simulink model "Rad_model"  (R2020a)
settings: Solver=VariableStepAuto  StartTime=0.0  StopTime=10.0  RelTol=1e-3
undefined symbols (not defined in the file or in its folder): paramRadarMT, phased, physconst
libraries: phaseddetectlib x5, phasedenvlib x4, phasedtxrxlib x4, simulink x1, phasedbflib x1, phasedwavlib x1, phaseddoalib x1
settings Model: Creator=saini  LastModifiedBy=saini

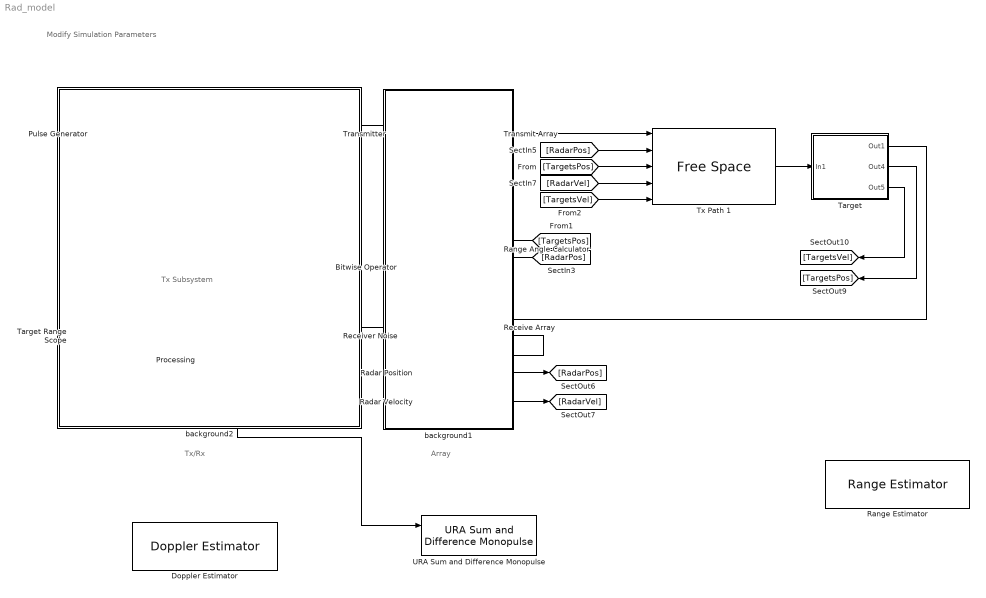
== system Rad_model ==
  note: Modify Simulation Parameters
  note: Tx/Rx
  note: Tx Subsystem
  note: Array
  Bitwise Operator : simulink/Logic and Bit Operations/Bitwise Operator  logicop=NOT  UseBitMask=off  BitMask=bin2dec('11011001')  BitMaskRealWorld=Stored Integer
  Doppler Estimator : phaseddetectlib/Doppler Estimator  NumEstimatesSource=Property  NumEstimates=1  VarianceOutputPort=off  NumPulses=2  NoisePowerSource=Property  NoisePower=1  ClusterInputPort=off  SimulateUsing=Interpreted execution
      settings: SourceProductBaseCode=AR
  Processing : Subsystem
      mask Display: disp('Signal Processing')
  Pulse Generator : phasedwavlib/Rectangular Waveform  SampleRate=paramRadarMT.fs  DurationSpecification=Pulse width  PulseWidth=1/paramRadarMT.pulseBw  DutyCycle=0.5  PRF=paramRadarMT.prf  PRFSelectionInputPort=off  SimulationTimeSource=Derive from waveform parameters  OutputFormat=Pulses  NumSamples=100  NumPulses=1  PRFOutputPort=off  SimulateUsing=Interpreted execution
      settings: SourceProductBaseCode=AR
  Radar Position : Constant  Value=[ 0; 0; 0 ]  SampleTime=1/paramRadarMT.prf
  Radar Velocity : Constant  Value=[ 0; 0; 0 ]  SampleTime=1/paramRadarMT.prf
  Range Angle Calculator : phasedenvlib/Range Angle Calculator  Model=Free space  ReferencePositionSource=Input port  ReferencePosition=[ 0; 0; 0 ]  ReferenceAxesSource=Property  ReferenceAxes=eye( 3 )  Output=Angle  SimulateUsing=Interpreted execution
      settings: SourceProductBaseCode=AR
  Range Estimator : phaseddetectlib/Range Estimator  NumEstimatesSource=Property  NumEstimates=1  VarianceOutputPort=off  RMSResolution=1  NoisePowerSource=Property  NoisePower=1  ClusterInputPort=off  SimulateUsing=Interpreted execution
      settings: SourceProductBaseCode=AR
  Receive Array : phasedtxrxlib/Narrowband Receive Array  PropagationSpeed=paramRadarMT.propSpeed  OperatingFrequency=paramRadarMT.fc  Wavefront=Plane  SensorGainMeasure=dB  Polarization=None  WeightsInputPort=off  SimulateUsing=Interpreted execution  Sensor=phased.URA('ElementSpacing',0.0150,'Size',[ 5, 5 ],'Element',phased.IsotropicAntennaElement('FrequencyRange',[ 5e9, 15e9 ]))
      settings: SourceProductBaseCode=AR
  Receiver Noise : phasedtxrxlib/Receiver Preamp  Gain=20  LossFactor=0  NoiseMethod=Noise temperature  NoiseFigure=0  ReferenceTemperature=290  SampleRateFromInputCheckbox=on  SampleRate=1e6  NoisePower=0  EnableInputPort=on  PhaseNoiseInputPort=off  SeedSource=Auto  Seed=0  SimulateUsing=Interpreted execution
      settings: SourceProductBaseCode=AR
  Target : Subsystem
      mask Display:
      | disp('Targets')
      | port_label('input',1,'X');
      | port_label('output',1,'Y');
      | port_label('output',2,'Pos');
      | port_label('output',3,'Vel');
  Target Range Scope : ArrayPlot
  Transmit Array : phasedtxrxlib/Narrowband Transmit Array  PropagationSpeed=paramRadarMT.propSpeed  OperatingFrequency=paramRadarMT.fc  CombineRadiatedSignals=on  SensorGainMeasure=dB  Polarization=None  WeightsInputPort=off  SimulateUsing=Interpreted execution  Sensor=phased.URA('Size',[ 5, 5 ],'ElementSpacing',0.0150,'Element',phased.IsotropicAntennaElement('FrequencyRange',[ 5e9, 15e9 ]))
      settings: SourceProductBaseCode=AR
  Transmitter : phasedtxrxlib/Transmitter  PeakPower=paramRadarMT.peakPower/16  Gain=paramRadarMT.txGain  LossFactor=0  InUseOutputPort=on  CoherentOnTransmit=on  PhaseNoiseOutputPort=off  SeedSource=Auto  Seed=0  SimulateUsing=Interpreted execution
      settings: SourceProductBaseCode=AR
  Tx Path 1 : phasedenvlib/Free Space  PropagationSpeed=paramRadarMT.propSpeed  OperatingFrequency=paramRadarMT.fc  TwoWayPropagation=on  SampleRateFromInputCheckbox=on  SampleRate=1e6  MaximumDistanceSource=Property  MaximumDistance=10e3  MaximumNumInputSamplesSource=Auto  MaximumNumInputSamples=1000  SimulateUsing=Interpreted execution
      settings: SourceProductBaseCode=AR
  URA Sum and Difference Monopulse : phaseddoalib/URA Sum and Difference Monopulse  PropagationSpeed=physconst( 'LightSpeed' )  OperatingFrequency=10e8  NumPhaseShifterBits=0  SimulateUsing=Interpreted execution  SensorArray=phased.URA('Element',phased.IsotropicAntennaElement('FrequencyRange',[ 5e9, 15e9 ]),'Size',[ 5, 5 ],'ElementSpacing',0.0150)
      settings: SourceProductBaseCode=AR
  background1 : Subsystem  Description=Jammer
      mask Display: disp('')
  background2 : Subsystem  Description=Jammer
      mask Display: disp('')
  wires:
  Target/1(Out1) -> Receive Array/1
  Target/3(Out5) -> [TargetsVel]
  [TargetsPos] -> Range Angle Calculator/1
  Tx Path 1/1 -> Target/1(In1)
  Target/2(Out4) -> [TargetsPos]
  [TargetsPos] -> Tx Path 1/3
  [TargetsVel] -> Tx Path 1/5
  [RadarVel] -> Tx Path 1/4
  Radar Velocity/1 -> [RadarVel]
  Transmitter/2 -> Bitwise Operator/1
  Processing/1(Out1) -> Target Range Scope/1
  Receiver Noise/1 -> URA Sum and Difference Monopulse/1, Processing/1(In1)
  Range Angle Calculator/1 -> Receive Array/2, Transmit Array/2
  Transmit Array/1 -> Tx Path 1/1
  [RadarPos] -> Range Angle Calculator/2
  [RadarPos] -> Tx Path 1/2
  Receive Array/1 -> Receiver Noise/1
  Radar Position/1 -> [RadarPos]
  Bitwise Operator/1 -> Receiver Noise/2
  Transmitter/1 -> Transmit Array/1
  Pulse Generator/1 -> Transmitter/1

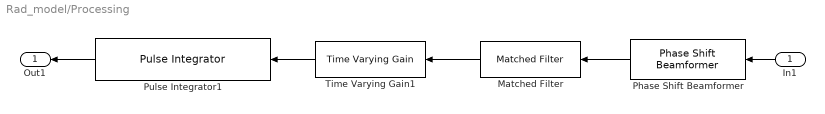
== system Rad_model/Processing ==
  In1 : Inport
  Matched Filter : phaseddetectlib/Matched Filter  CoefficientsSource=Property  Coefficients=paramRadarMT.matchingCoeff  SpectrumWindow=None  CustomSpectrumWindow=@hamming  SpectrumRange=[ 0, 1e5 ]  SampleRateFromInputCheckbox=on  SampleRate=1e6  SidelobeAttenuation=30  Beta=0.5  Nbar=4  GainOutputPort=off  MaximumNumInputSamplesSource=Auto  MaximumNumInputSamples=100  SimulateUsing=Interpreted execution
      settings: SourceProductBaseCode=AR
  Phase Shift Beamformer : phasedbflib/Phase Shift Beamformer  PropagationSpeed=paramRadarMT.propSpeed  OperatingFrequency=paramRadarMT.fc  DirectionSource=Property  Direction=[ 0; 0 ]  NumPhaseShifterBits=0  WeightsNormalization=Distortionless  WeightsOutputPort=off  SimulateUsing=Interpreted execution  SensorArray=phased.URA('ElementSpacing',0.0150,'Size',[ 5, 5 ],'Element',phased.IsotropicAntennaElement('FrequencyRange',[ 5e9, 15e9 ]))
      settings: SourceProductBaseCode=AR
  Pulse Integrator1 : phaseddetectlib/Pulse Integrator  CoherentFlag=Noncoherent  N=10  V=0
      settings: SourceProductBaseCode=AR
  Time Varying Gain1 : phaseddetectlib/Time Varying Gain  RangeLossSource=Property  RangeLoss=paramRadarMT.rangeLoss  ReferenceLoss=paramRadarMT.referenceLoss  SimulateUsing=Interpreted execution
      settings: SourceProductBaseCode=AR
  Out1 : Outport  VectorParamsAs1DForOutWhenUnconnected=off
  wires:
  Time Varying Gain1/1 -> Pulse Integrator1/1
  Matched Filter/1 -> Time Varying Gain1/1
  Pulse Integrator1/1 -> Out1/1
  In1/1 -> Phase Shift Beamformer/1
  Phase Shift Beamformer/1 -> Matched Filter/1

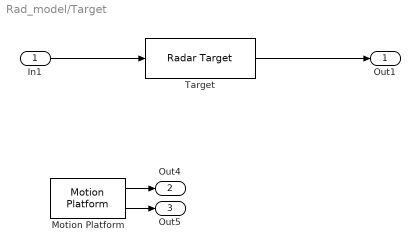
== system Rad_model/Target ==
  In1 : Inport
  Motion Platform : phasedenvlib/Motion Platform  MotionModel=Velocity  InitialPosition=paramRadarMT.targetPos  InitialVelocity=[ 0; 0; 0 ]  VelocitySource=Property  Velocity=paramRadarMT.targetVel  AccelerationSource=Property  Acceleration=[0;0;0]  CustomTrajectory=[ 0, 0, 0, 0, 0, 0, 0; 1, 0, 0, 0, 0, 0, 0 ]  ScanMode=None  InitialScanAngle=0  AzimuthSpan=[ -60, 60 ]  AzimuthScanRate=10  InitialOrientationAxes=eye(3)  OrientationAxesOutputPort=off  ElapsedTimeSource=Auto  SampleRateFromInputCheckbox=on  SampleRate=1e6  SimulateUsing=Interpreted execution
      settings: SourceProductBaseCode=AR
  Target : phasedenvlib/Radar Target  EnablePolarization=off  Mode=Monostatic  MeanRCSSource=Property  ScatteringMatrixSource=Property  MeanRCS=paramRadarMT.targetRcs  ScatteringMatrix=eye( 2 )  Model=Nonfluctuating  PropagationSpeed=paramRadarMT.propSpeed  OperatingFrequency=paramRadarMT.fc  SeedSource=Auto  Seed=0  SimulateUsing=Interpreted execution
      settings: SourceProductBaseCode=AR
  Out1 : Outport  VectorParamsAs1DForOutWhenUnconnected=off
  Out4 : Outport  Port=2  VectorParamsAs1DForOutWhenUnconnected=off
  Out5 : Outport  Port=3  VectorParamsAs1DForOutWhenUnconnected=off
  wires:
  In1/1 -> Target/1
  Target/1 -> Out1/1
  Motion Platform/1 -> Out4/1
  Motion Platform/2 -> Out5/1

== system Rad_model/background1 ==

== system Rad_model/background2 ==
